simulink model "Zadanie_M3b"  (R2021b)
settings: Solver=VariableStepAuto  StartTime=0.0  StopTime=10.0  MaxStep=0.01  RelTol=1e-3
settings Model: Creator=Studenci  LastModifiedBy=Studenci

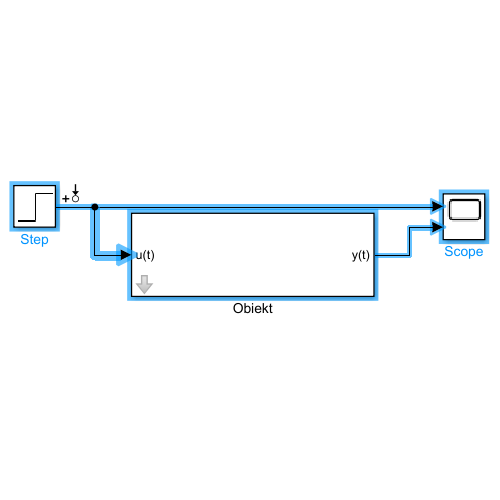
[thumbnail: Simulink's stored preview of the top-level diagram]
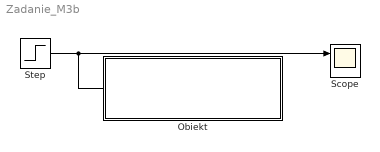
== system Zadanie_M3b ==
  Obiekt : Subsystem  mask{wn=1, zeta=0.5}
      mask prompts: wn "wn - częstotliwość drgań własnych"; zeta "zeta - współczynnik tłumienia"
  Scope : Scope  NumInputPorts=2
  Step : Step  Time=0  SampleTime=0
  wires:
  ? -> Scope/2
  Step/1 -> Scope/1

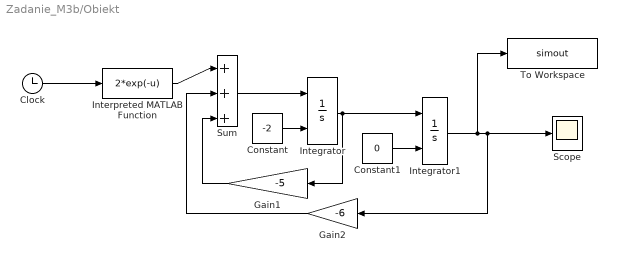
== system Zadanie_M3b/Obiekt ==
  Clock : Clock
  Constant : Constant  Value=-2
  Constant1 : Constant  Value=0
  Gain1 : Gain  Gain=-5
  Gain2 : Gain  Gain=-6
  Integrator : Integrator  InitialConditionSource=external
  Integrator1 : Integrator  InitialConditionSource=external
  Interpreted MATLAB Function : MATLABFcn  MATLABFcn=2*exp(-u)
  Scope : Scope
  Sum : Sum  Inputs=|+++
  To Workspace : ToWorkspace  VariableName=simout  SaveFormat=Timeseries  SampleTime=-1
  wires:
  Constant/1 -> Integrator/2
  Sum/1 -> Integrator/1
  Integrator/1 -> Gain1/1, Integrator1/1
  Constant1/1 -> Integrator1/2
  Integrator1/1 -> To Workspace/1, Scope/1, Gain2/1
  Gain1/1 -> Sum/3
  Gain2/1 -> Sum/2
  Interpreted MATLAB Function/1 -> Sum/1
  Clock/1 -> Interpreted MATLAB Function/1
